simulink model "N_phase_two_level_inverter"  (R2021a)
settings: Solver=ode4  StartTime=0.0  StopTime=0.5  FixedStep=1e-6  RelTol=1e-3
libraries: spsIGBTDiodeLib x18, spsCurrentMeasurementLib x9, spsSeriesRLCBranchLib x9, spsVoltageMeasurementLib x9, spsGroundLib x3, spsDCVoltageSourceLib x2, simulink x1, spspowerguiLib x1
settings Model: Creator=PRANAY KAMAL  LastModifiedBy=PRANAY KAMAL
settings DataIOCC: ReturnWorkspaceOutputs=off

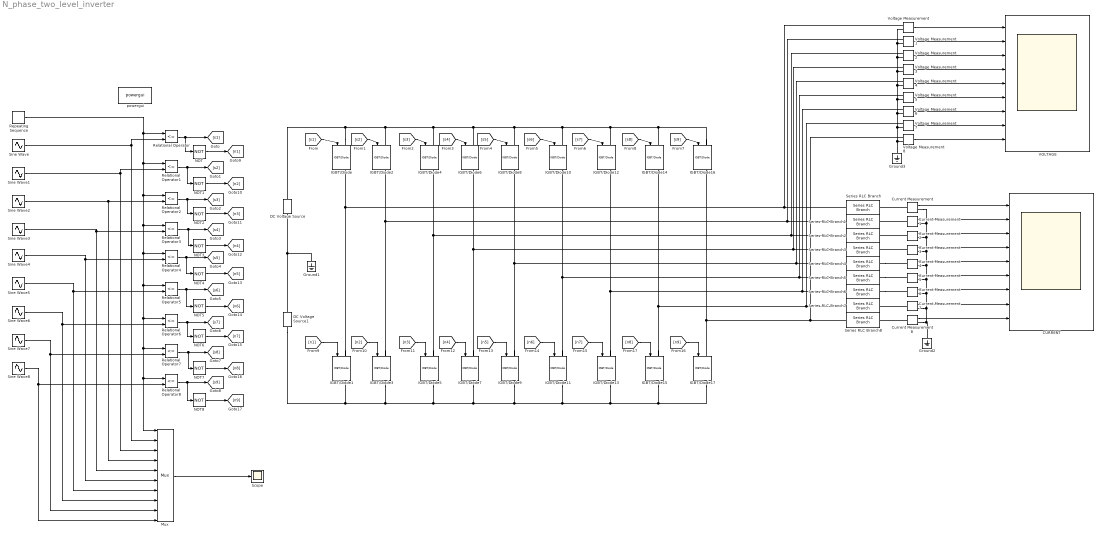
== system N_phase_two_level_inverter ==
  CURRENT : Scope  NumInputPorts=9
  Current Measurement{,1..8} (9 alike) : spsCurrentMeasurementLib/Current Measurement  PhasorSimulation=off  OutputType=Complex  PSBequivalent=0
  DC Voltage Source : spsDCVoltageSourceLib/DC Voltage Source  Amplitude=100  Measurements=None
  DC Voltage Source1 : spsDCVoltageSourceLib/DC Voltage Source  Amplitude=100  Measurements=None
  Ground1 : spsGroundLib/Ground  LConnTagsString=a
  Ground2 : spsGroundLib/Ground  LConnTagsString=a
  Ground3 : spsGroundLib/Ground  LConnTagsString=a
  IGBT/Diode{,1..17} (18 alike) : spsIGBTDiodeLib/IGBT//Diode  Ron=1e-3  Rs=1e5  Cs=inf  Measurements=on
  Mux : Mux  Inputs=10
  NOT{,1..8} (9 alike) : Logic  Operator=NOT  IconShape=distinctive  AllPortsSameDT=off  OutDataTypeStr=boolean
  Relational Operator{,1..8} (9 alike) : RelationalOperator  Operator=<=  OutDataTypeStr=boolean  RndMeth=Simplest
  Repeating Sequence : simulink/Sources/Repeating Sequence  rep_seq_t=[0 0.5 1]*(1/5000)  rep_seq_y=[1 -1 1]
  Scope : Scope
  Series RLC Branch{,1..8} (9 alike) : spsSeriesRLCBranchLib/Series RLC Branch  LConnTagsString=__new0  RConnTagsString=__new0  BranchType=RL  Resistance=0.1  Inductance=1e-2  SetiL0=off  InitialCurrent=0  Capacitance=1e-6  Setx0=off  InitialVoltage=0  Measurements=None
  Sine Wave : Sin  Frequency=2*pi*50  SampleTime=0
  Sine Wave1 : Sin  Frequency=2*pi*50  Phase=2*pi/9  SampleTime=0
  Sine Wave2 : Sin  Frequency=2*pi*50  Phase=4*pi/9  SampleTime=0
  Sine Wave3 : Sin  Frequency=2*pi*50  Phase=2*pi/3  SampleTime=0
  Sine Wave4 : Sin  Frequency=2*pi*50  Phase=8*pi/9  SampleTime=0
  Sine Wave5 : Sin  Frequency=2*pi*50  Phase=10*pi/9  SampleTime=0
  Sine Wave6 : Sin  Frequency=2*pi*50  Phase=4*pi/3  SampleTime=0
  Sine Wave7 : Sin  Frequency=2*pi*50  Phase=14*pi/9  SampleTime=0
  Sine Wave8 : Sin  Frequency=2*pi*50  Phase=16*pi/9  SampleTime=0
  VOLTAGE : Scope  NumInputPorts=9
  Voltage Measurement{,1..8} (9 alike) : spsVoltageMeasurementLib/Voltage Measurement  PhasorSimulation=off  OutputType=Complex  PSBequivalent=0
  powergui : spspowerguiLib/powergui  Priority=1  SimulationMode=Continuous  SampleTime=50e-6  frequency=60  Iterations=50  frequencyindice=0  Pbase=100e6  ErrMax=1e-4  UnitsV=kV  UnitsW=MW  buscounter=0  FunctionMessages=off  echomessages=off  EnableUseOfTLC=off  CurrentSourceSwitches=off  DisableSnubberDevices=off  DisableRonSwitches=off  DisableVfSwitches=off  DisplayEquations=off  AutomaticDiscreteSolvers=off  SolverType=Tustin/Backward Euler (TBE)  Interpol=off  ExternalGateDelay=off  methode=off  Ts=100  x0status=blocks  SPID=on  SwTol=0  HookPort=off  NonlinearTolerance=1e-4  nMaxIteration=100  ContinueOnMaxIteration=off  RestoreLinks=warning  ResistiveCurrentMeasurement=off  Frange=[0:2:500]  Ylog=off  Xlog=on  ShowGrid=off  save=off  variable=ZData  structure=0  ZoomFFT=off  StartTime=0.0  cycles=1  DisplayStyle=1  fundamental=60  FreqAxis=off  MaxFrequency=1000  frequencyindicesteady=1  RmsSteady=1  display=off
  wires:
  Mux/1 -> Scope/1
  Repeating Sequence/1 -> Relational Operator/1, Relational Operator1/1, Relational Operator2/1, Relational Operator3/1, Relational Operator4/1, Relational Operator5/1, Relational Operator7/1, Relational Operator8/1, Mux/1, Relational Operator6/1
  Sine Wave/1 -> Relational Operator/2, Mux/2
  Sine Wave1/1 -> Relational Operator1/2, Mux/3
  Sine Wave3/1 -> Relational Operator3/2, Mux/5
  Sine Wave4/1 -> Relational Operator4/2, Mux/6
  Sine Wave5/1 -> Relational Operator5/2, Mux/7
  Sine Wave6/1 -> Relational Operator6/2, Mux/8
  Sine Wave7/1 -> Relational Operator7/2, Mux/9
  Sine Wave8/1 -> Relational Operator8/2, Mux/10
  Sine Wave2/1 -> Relational Operator2/2, Mux/4
  Relational Operator/1 -> NOT/1, [s1]
  Relational Operator1/1 -> NOT1/1, [s2]
  Relational Operator2/1 -> NOT2/1, [s3]
  Relational Operator3/1 -> NOT3/1, [s4]
  Relational Operator4/1 -> NOT4/1, [s5]
  Relational Operator5/1 -> NOT5/1, [s6]
  Relational Operator6/1 -> NOT6/1, [s7]
  Relational Operator7/1 -> NOT7/1, [s8]
  Relational Operator8/1 -> NOT8/1, [s9]
  [s1] -> IGBT/Diode/1
  [s2] -> IGBT/Diode2/1
  [s3] -> IGBT/Diode4/1
  [s4] -> IGBT/Diode6/1
  [s5] -> IGBT/Diode8/1
  [s6] -> IGBT/Diode10/1
  [s7] -> IGBT/Diode12/1
  [s8] -> IGBT/Diode14/1
  [s9] -> IGBT/Diode16/1
  NOT/1 -> [n1]
  NOT1/1 -> [n2]
  NOT2/1 -> [n3]
  NOT3/1 -> [n4]
  NOT4/1 -> [n5]
  NOT5/1 -> [n6]
  NOT8/1 -> [n9]
  NOT7/1 -> [n8]
  NOT6/1 -> [n7]
  [n1] -> IGBT/Diode1/1
  [n2] -> IGBT/Diode3/1
  [n3] -> IGBT/Diode5/1
  [n4] -> IGBT/Diode7/1
  [n5] -> IGBT/Diode9/1
  [n6] -> IGBT/Diode11/1
  [n7] -> IGBT/Diode13/1
  [n8] -> IGBT/Diode15/1
  [n9] -> IGBT/Diode17/1
  Voltage Measurement/1 -> VOLTAGE/1
  Voltage Measurement1/1 -> VOLTAGE/2
  Voltage Measurement3/1 -> VOLTAGE/4
  Voltage Measurement2/1 -> VOLTAGE/3
  Voltage Measurement4/1 -> VOLTAGE/5
  Voltage Measurement5/1 -> VOLTAGE/6
  Voltage Measurement8/1 -> VOLTAGE/9
  Voltage Measurement7/1 -> VOLTAGE/8
  Voltage Measurement6/1 -> VOLTAGE/7
  Current Measurement4/1 -> CURRENT/5
  Current Measurement8/1 -> CURRENT/9
  Current Measurement6/1 -> CURRENT/7
  Current Measurement7/1 -> CURRENT/8
  Current Measurement3/1 -> CURRENT/4
  Current Measurement5/1 -> CURRENT/6
  Current Measurement1/1 -> CURRENT/2
  Current Measurement2/1 -> CURRENT/3
  Current Measurement/1 -> CURRENT/1
  connections:
  IGBT/Diode/LConn1 -- DC Voltage Source/RConn1 -- IGBT/Diode16/LConn1 -- IGBT/Diode14/LConn1 -- IGBT/Diode12/LConn1 -- IGBT/Diode10/LConn1 -- IGBT/Diode8/LConn1 -- IGBT/Diode6/LConn1 -- IGBT/Diode4/LConn1 -- IGBT/Diode2/LConn1
  IGBT/Diode3/RConn1 -- IGBT/Diode17/RConn1 -- IGBT/Diode15/RConn1 -- IGBT/Diode13/RConn1 -- IGBT/Diode11/RConn1 -- IGBT/Diode9/RConn1 -- IGBT/Diode7/RConn1 -- IGBT/Diode5/RConn1 -- DC Voltage Source1/LConn1 -- IGBT/Diode1/RConn1
  IGBT/Diode1/LConn1 -- Voltage Measurement/LConn1 -- Series RLC Branch/LConn1 -- IGBT/Diode/RConn1
  IGBT/Diode3/LConn1 -- Voltage Measurement1/LConn1 -- Series RLC Branch1/LConn1 -- IGBT/Diode2/RConn1
  IGBT/Diode5/LConn1 -- Voltage Measurement2/LConn1 -- Series RLC Branch2/LConn1 -- IGBT/Diode4/RConn1
  IGBT/Diode7/LConn1 -- Voltage Measurement3/LConn1 -- Series RLC Branch3/LConn1 -- IGBT/Diode6/RConn1
  IGBT/Diode9/LConn1 -- Voltage Measurement4/LConn1 -- Series RLC Branch4/LConn1 -- IGBT/Diode8/RConn1
  IGBT/Diode11/LConn1 -- Voltage Measurement5/LConn1 -- Series RLC Branch5/LConn1 -- IGBT/Diode10/RConn1
  IGBT/Diode13/LConn1 -- Voltage Measurement6/LConn1 -- Series RLC Branch6/LConn1 -- IGBT/Diode12/RConn1
  IGBT/Diode15/LConn1 -- Voltage Measurement7/LConn1 -- Series RLC Branch7/LConn1 -- IGBT/Diode14/RConn1
  IGBT/Diode17/LConn1 -- Voltage Measurement8/LConn1 -- Series RLC Branch8/LConn1 -- IGBT/Diode16/RConn1
  DC Voltage Source1/RConn1 -- Ground1/LConn1 -- DC Voltage Source/LConn1
  Current Measurement/LConn1 -- Series RLC Branch/RConn1
  Current Measurement1/LConn1 -- Series RLC Branch1/RConn1
  Current Measurement2/LConn1 -- Series RLC Branch2/RConn1
  Current Measurement3/LConn1 -- Series RLC Branch3/RConn1
  Current Measurement7/LConn1 -- Series RLC Branch7/RConn1
  Series RLC Branch6/RConn1 -- Current Measurement6/LConn1
  Series RLC Branch5/RConn1 -- Current Measurement5/LConn1
  Series RLC Branch4/RConn1 -- Current Measurement4/LConn1
  Current Measurement8/LConn1 -- Series RLC Branch8/RConn1
  Current Measurement/RConn1 -- Ground2/LConn1 -- Current Measurement8/RConn1 -- Current Measurement7/RConn1 -- Current Measurement6/RConn1 -- Current Measurement5/RConn1 -- Current Measurement4/RConn1 -- Current Measurement3/RConn1 -- Current Measurement2/RConn1 -- Current Measurement1/RConn1
  Voltage Measurement8/LConn2 -- Ground3/LConn1 -- Voltage Measurement/LConn2 -- Voltage Measurement1/LConn2 -- Voltage Measurement2/LConn2 -- Voltage Measurement3/LConn2 -- Voltage Measurement4/LConn2 -- Voltage Measurement5/LConn2 -- Voltage Measurement6/LConn2 -- Voltage Measurement7/LConn2
